simulink model "B2"  (R2022b)
settings: Solver=VariableStepAuto  StartTime=0.0  StopTime=40  RelTol=1e-3
settings Model: Creator=Asus  LastModifiedBy=Asus

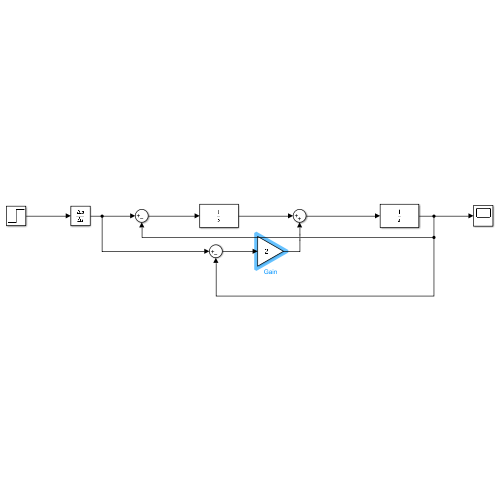
[thumbnail: Simulink's stored preview of the top-level diagram]
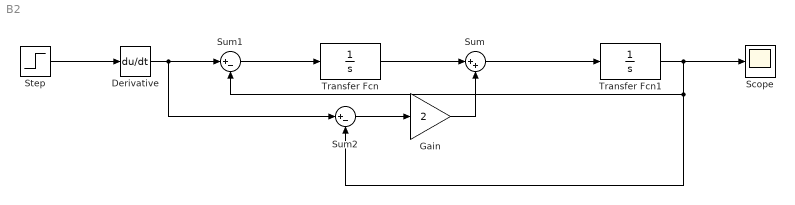
== system B2 ==
  Derivative : Derivative
  Gain : Gain  Gain=2
  Scope : Scope
  Step : Step  SampleTime=0
  Sum : Sum  Inputs=|++
  Sum1 : Sum  Inputs=|+-
  Sum2 : Sum  Inputs=|+-
  Transfer Fcn : TransferFcn  Denominator=[1 0]
  Transfer Fcn1 : TransferFcn  Denominator=[1 0]
  wires:
  Transfer Fcn/1 -> Sum/1
  Sum/1 -> Transfer Fcn1/1
  Sum1/1 -> Transfer Fcn/1
  Transfer Fcn1/1 -> Scope/1, Sum1/2, Sum2/2
  Gain/1 -> Sum/2
  Sum2/1 -> Gain/1
  Step/1 -> Derivative/1
  Derivative/1 -> Sum2/1, Sum1/1
